simulink model "Workforcedistance_1640261450"  (R2021b)
settings: Solver=VariableStepAuto  StartTime=0.0  StopTime=50.0  RelTol=1e-3
undefined symbols (not defined in the file or in its folder): sigbuilder_block
settings Model: Creator=Ish  LastModifiedBy=Ish

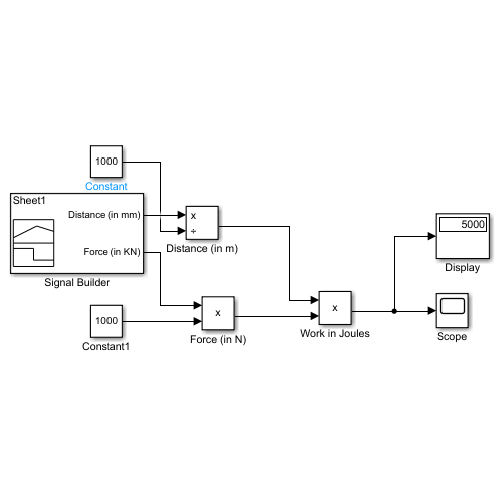
[thumbnail: Simulink's stored preview of the top-level diagram]
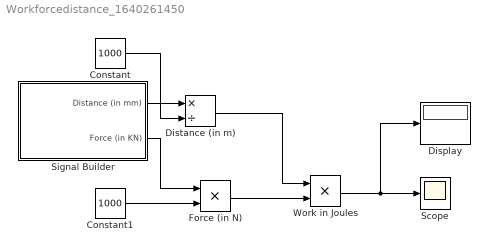
== system Workforcedistance_1640261450 ==
  Constant : Constant  Value=1000
  Constant1 : Constant  Value=1000
  Display : Display
  Distance (in m) : Product  Inputs=*/
  Force (in N) : Product
  Scope : Scope
  Signal Builder : Subsystem  Tag=STV Subsys  LoadFcn=sigbuilder_block('load');  StartFcn=sigbuilder_block('start');  StopFcn=sigbuilder_block('stop');  ClipboardFcn=sigbuilder_block('clipboard');  mask(Sigbuilder block){tuvar=[0:10]}
      mask help: Simulink:masks:SigbuilderBlock_MD
      mask init:
      | if ~strcmp(get_param(bdroot(gcbh),'SimulationStatus'),'stopped') tuvar = sigbuilder_block('maskInit'); end
      settings: CopyFcn=sigbuilder_block('copy');  DeleteFcn=sigbuilder_block('delete');  ModelCloseFcn=sigbuilder_block('modelClose');  PreSaveFcn=sigbuilder_block('preSave');  PauseFcn=sigbuilder_block('pause');  ContinueFcn=sigbuilder_block('continue');  NameChangeFcn=sigbuilder_block('namechange');  OpenFcn=sigbuilder_block('open',[437.6 153 550.4 359.25 ]);  CloseFcn=sigbuilder_block('close');
      mask Display: plot(0, 0, 100, 100,[2, 2, 32, 32, 2], [68, 8, 8, 68, 68],[32, 2], [38, 38], [32, 19, 2],[53, 60, 44], [32, 17, 17, 2],[16, 16, 31, 31]);txt = getActiveGroup(gcbh);text(2, 100, txt,'verticalAlignment', 'top');
  Work in Joules : Product
  wires:
  Distance (in m)/1 -> Work in Joules/1
  Force (in N)/1 -> Work in Joules/2
  Constant1/1 -> Force (in N)/2
  Constant/1 -> Distance (in m)/2
  Signal Builder/2(Force (in KN)) -> Force (in N)/1
  Signal Builder/1(Distance (in mm)) -> Distance (in m)/1
  Work in Joules/1 -> Scope/1, Display/1

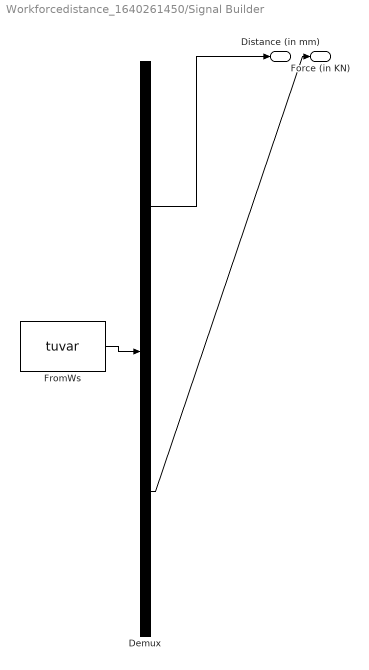
== system Workforcedistance_1640261450/Signal Builder ==
  Demux : Demux  Tag=STV Demux  Outputs=2
      settings: DisplayOption=none
  FromWs : FromWorkspace  Tag=STV FromWs  VariableName=tuvar
      SigBuilderData=|
      | common.afterFinalStr = 'Extrapolate'
      | common.sampleTime = 0
      | dataSet.timeRange = [0 50]
      | dataSet.name = 'Sheet1'
      | sbobj.Groups.Name = 'Sheet1'
      | sbobj.Groups.Signals(1).Name = 'Distance (in mm)'
      | sbobj.Groups.Signals(1).XData = [0 10 20 30 40 50]
      | sbobj.Groups.Signals(1).YData = [0 20 40 60 80 100]
      | sbobj.Groups.Signals(2).Name = 'Force (in KN)'
      | sbobj.Groups.Signals(2).XData = [0 10 20 30 40 50]
      | sbobj.Groups.Signals(2).YData = [60 72 65 53 44 50]
      | sbobj.Groups.TimeRange = [0 50]
  Distance (in mm) : Outport  Tag=STV Outport
  Force (in KN) : Outport  Tag=STV Outport  Port=2
  wires:
  Demux/1 -> Distance (in mm)/1
  FromWs/1 -> Demux/1
  Demux/2 -> Force (in KN)/1
